simulink model "admire_linear_test"  (Simulink 3.00)
settings: Solver=ode4  StartTime=0.0  StopTime=30  FixedStep=0.008  RelTol=1e-3
undefined symbols (not defined in the file or in its folder): Abare, Afcs, Alt, Bbare, Bfcs, Cbare, Cfcs, dalt_err, Dbare, ddc_bw, ddc_rate, ddei_bw, ddei_rate, ddey_bw, ddey_rate, ddle_bw, ddle_rate, ddr_bw, ddr_rate, Dfcs, dMach_err, Mach, rlimit_c, rlimit_ie, rlimit_le, rlimit_oe, rlimit_r, y0bare
libraries: simulink_extras x16
settings Model: TimeSaveName=tout_lin  OutputSaveName=yout_lin  LastModifiedBy=hkg

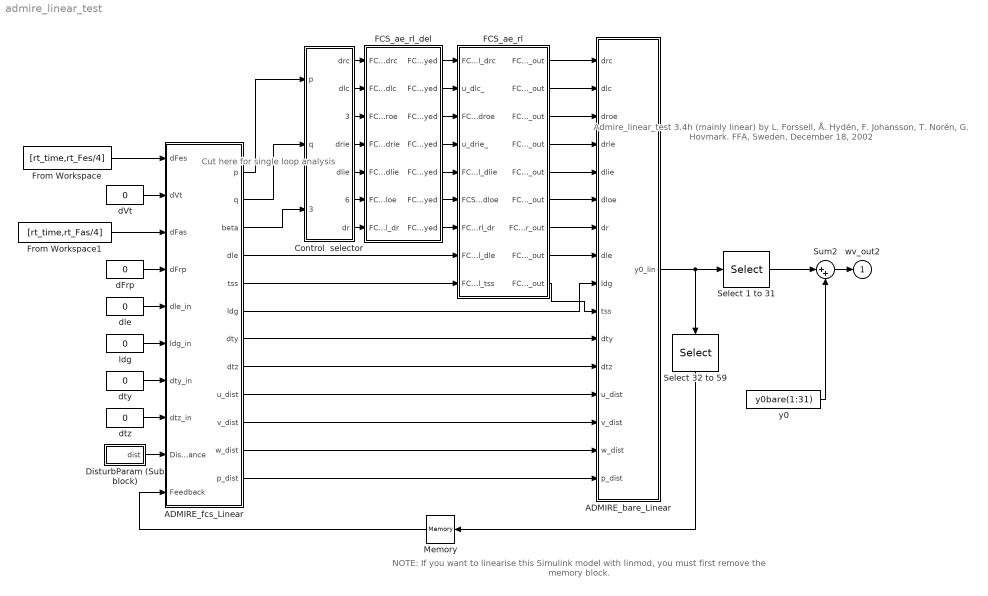
== system admire_linear_test ==
  note: Admire_linear_test 3.4h
      | (mainly linear)
      | by  L. Forssell,
      | Å. Hydén,
      | F. Johansson,
      | T. Norén,
      | G. Hovmark.
      | FFA, Sweden,
      | December 18, 2002
  note: Cut
      | here
      | for
      | single
      | loop
      | analysis
  note: NOTE: If you want to linearise this Simulink model
      | with linmod, you must first
      | remove the memory block.
  ADMIRE_bare_Linear : Subsystem
  ADMIRE_fcs_Linear : Subsystem
  Control  selector : Subsystem
  DisturbParam (Sub block) : Subsystem
  FCS_ae_rl : Subsystem
      mask Display: disp('Saturators,\nRatelimiters\nand\nActuators\n\nMach No and\nrate limiter\ndata are\ntaken from\nWorkspace\n\nAll inital\nstates empty')
  FCS_ae_rl_del : Subsystem
      mask Display: disp('Total\nComputer\nDelay\n\nAll inital\nstates empty')
  From Workspace : FromWorkspace  VariableName=[rt_time,rt_Fes/4]  SampleTime=0  HoldFinalValue=off
  From Workspace1 : FromWorkspace  VariableName=[rt_time,rt_Fas/4]  SampleTime=0  HoldFinalValue=off
  Memory : Memory  Orientation=left  X0=0  InheritSampleTime=off
  Select 1 to 31 : Selector  Elements=[1:31]  InputPortWidth=59
  Select 32 to 59 : Selector  Orientation=down  Elements=[32:59]  InputPortWidth=59
  Sum2 : Sum  Inputs=|++  SaturateOnIntegerOverflow=on
  dFrp : Constant  Value=0
  dVt : Constant  Value=0
  dle : Constant  Value=0
  dty : Constant  Value=0
  dtz : Constant  Value=0
  ldg : Constant  Value=0
  y0 : Constant  Value=y0bare(1:31)
  wv_out2 : Outport  Port=1  InitialOutput=0
  wires:
  dle/1 -> ADMIRE_fcs_Linear/5(dle_in)
  ldg/1 -> ADMIRE_fcs_Linear/6(ldg_in)
  dty/1 -> ADMIRE_fcs_Linear/7(dty_in)
  dtz/1 -> ADMIRE_fcs_Linear/8(dtz_in)
  DisturbParam (Sub block)/1(dist) -> ADMIRE_fcs_Linear/9(Disturbance)
  dFrp/1 -> ADMIRE_fcs_Linear/4(dFrp)
  dVt/1 -> ADMIRE_fcs_Linear/2(dVt)
  ADMIRE_fcs_Linear/12(p_dist) -> ADMIRE_bare_Linear/16(p_dist)
  ADMIRE_fcs_Linear/8(dtz) -> ADMIRE_bare_Linear/12(dtz)
  ADMIRE_fcs_Linear/7(dty) -> ADMIRE_bare_Linear/11(dty)
  FCS_ae_rl_del/1(FCS_ae_rl_del_drc_delayed) -> FCS_ae_rl/1(FCS_ae_rl_drc)
  FCS_ae_rl_del/2(FCS_ae_rl_del_dlc_delayed) -> FCS_ae_rl/2(u_dlc_)
  FCS_ae_rl_del/3(FCS_ae_rl_del_droe_delayed) -> FCS_ae_rl/3(FCS_ae_rl_droe)
  FCS_ae_rl_del/4(FCS_ae_rl_del_drie_delayed) -> FCS_ae_rl/4(u_drie_)
  FCS_ae_rl_del/5(FCS_ae_rl_del_dlie_delayed) -> FCS_ae_rl/5(FCS_ae_rl_dlie)
  FCS_ae_rl_del/6(FCS_ae_rl_del_dloe_delayed) -> FCS_ae_rl/6(FCS_ae_rl_dloe)
  FCS_ae_rl_del/7(FCS_ae_rl_del_dr_delayed) -> FCS_ae_rl/7(FCS_ae_rl_dr)
  ADMIRE_fcs_Linear/4(dle) -> FCS_ae_rl/8(FCS_ae_rl_dle)
  ADMIRE_fcs_Linear/5(tss) -> FCS_ae_rl/9(FCS_ae_rl_tss)
  ADMIRE_fcs_Linear/6(ldg) -> ADMIRE_bare_Linear/9(ldg)
  ADMIRE_fcs_Linear/9(u_dist) -> ADMIRE_bare_Linear/13(u_dist)
  ADMIRE_fcs_Linear/10(v_dist) -> ADMIRE_bare_Linear/14(v_dist)
  ADMIRE_fcs_Linear/11(w_dist) -> ADMIRE_bare_Linear/15(w_dist)
  FCS_ae_rl/1(FCS_ae_rl_drc_out) -> ADMIRE_bare_Linear/1(drc)
  FCS_ae_rl/2(FCS_ae_rl_dlc_out) -> ADMIRE_bare_Linear/2(dlc)
  FCS_ae_rl/3(FCS_ae_rl_droe_out) -> ADMIRE_bare_Linear/3(droe)
  FCS_ae_rl/4(FCS_ae_rl_drie_out) -> ADMIRE_bare_Linear/4(drie)
  FCS_ae_rl/5(FCS_ae_rl_dlie_out) -> ADMIRE_bare_Linear/5(dlie)
  FCS_ae_rl/6(FCS_ae_rl_dloe_out) -> ADMIRE_bare_Linear/6(dloe)
  FCS_ae_rl/7(FCS_ae_rl_dr_out) -> ADMIRE_bare_Linear/7(dr)
  FCS_ae_rl/8(FCS_ae_rl_dle_out) -> ADMIRE_bare_Linear/8(dle)
  FCS_ae_rl/9(FCS_ae_rl_tss_out) -> ADMIRE_bare_Linear/10(tss)
  ADMIRE_bare_Linear/1(y0_lin) -> Select 1 to 31/1, Select 32 to 59/1
  Select 32 to 59/1 -> Memory/1
  Sum2/1 -> wv_out2/1
  y0/1 -> Sum2/2
  Select 1 to 31/1 -> Sum2/1
  Memory/1 -> ADMIRE_fcs_Linear/10(Feedback)
  Control  selector/1(drc) -> FCS_ae_rl_del/1(FCS_ae_rl_del_drc)
  Control  selector/2(dlc) -> FCS_ae_rl_del/2(FCS_ae_rl_del_dlc)
  Control  selector/3(droe) -> FCS_ae_rl_del/3(FCS_ae_rl_del_droe)
  Control  selector/4(drie) -> FCS_ae_rl_del/4(FCS_ae_rl_del_drie)
  Control  selector/5(dlie) -> FCS_ae_rl_del/5(FCS_ae_rl_del_dlie)
  Control  selector/6(dloe) -> FCS_ae_rl_del/6(FCS_ae_rl_del_dloe)
  Control  selector/7(dr) -> FCS_ae_rl_del/7(FCS_ae_rl_del_dr)
  ADMIRE_fcs_Linear/1(p) -> Control  selector/1(p)
  ADMIRE_fcs_Linear/2(q) -> Control  selector/2(q)
  ADMIRE_fcs_Linear/3(beta) -> Control  selector/3(beta)
  From Workspace/1 -> ADMIRE_fcs_Linear/1(dFes)
  From Workspace1/1 -> ADMIRE_fcs_Linear/3(dFas)

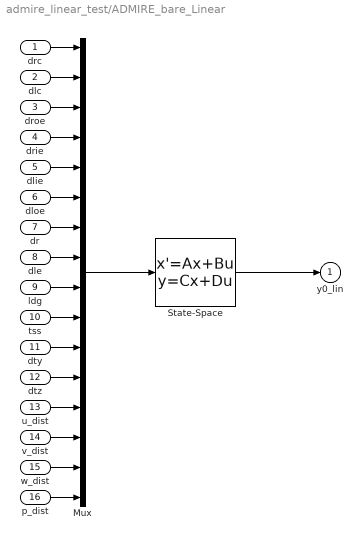
== system admire_linear_test/ADMIRE_bare_Linear ==
  drc : Inport  Port=1  PortWidth=-1  SampleTime=-1  DataType=auto
      settings: SignalType=auto
  dlc : Inport  Port=2  PortWidth=-1  SampleTime=-1  DataType=auto
      settings: SignalType=auto
  droe : Inport  Port=3  PortWidth=-1  SampleTime=-1  DataType=auto
      settings: SignalType=auto
  drie : Inport  Port=4  PortWidth=-1  SampleTime=-1  DataType=auto
      settings: SignalType=auto
  dlie : Inport  Port=5  PortWidth=-1  SampleTime=-1  DataType=auto
      settings: SignalType=auto
  dloe : Inport  Port=6  PortWidth=-1  SampleTime=-1  DataType=auto
      settings: SignalType=auto
  dr : Inport  Port=7  PortWidth=-1  SampleTime=-1  DataType=auto
      settings: SignalType=auto
  dle : Inport  Port=8  PortWidth=-1  SampleTime=-1  DataType=auto
      settings: SignalType=auto
  ldg : Inport  Port=9  PortWidth=-1  SampleTime=-1  DataType=auto
      settings: SignalType=auto
  tss : Inport  Port=10  PortWidth=-1  SampleTime=-1  DataType=auto
      settings: SignalType=auto
  dty : Inport  Port=11  PortWidth=-1  SampleTime=-1  DataType=auto
      settings: SignalType=auto
  dtz : Inport  Port=12  PortWidth=-1  SampleTime=-1  DataType=auto
      settings: SignalType=auto
  u_dist : Inport  Port=13  PortWidth=-1  SampleTime=-1  DataType=auto
      settings: SignalType=auto
  v_dist : Inport  Port=14  PortWidth=-1  SampleTime=-1  DataType=auto
      settings: SignalType=auto
  w_dist : Inport  Port=15  PortWidth=-1  SampleTime=-1  DataType=auto
      settings: SignalType=auto
  p_dist : Inport  Port=16  PortWidth=-1  SampleTime=-1  DataType=auto
      settings: SignalType=auto
  Mux : Mux  Inputs=16
      settings: DisplayOption=none
  State-Space : StateSpace  A=Abare  B=Bbare  C=Cbare  D=Dbare  X0=[]
  y0_lin : Outport  Port=1  InitialOutput=0
  wires:
  w_dist/1 -> Mux/15
  p_dist/1 -> Mux/16
  drc/1 -> Mux/1
  dlc/1 -> Mux/2
  droe/1 -> Mux/3
  drie/1 -> Mux/4
  dlie/1 -> Mux/5
  dloe/1 -> Mux/6
  dr/1 -> Mux/7
  dle/1 -> Mux/8
  ldg/1 -> Mux/9
  tss/1 -> Mux/10
  dty/1 -> Mux/11
  dtz/1 -> Mux/12
  u_dist/1 -> Mux/13
  v_dist/1 -> Mux/14
  Mux/1 -> State-Space/1
  State-Space/1 -> y0_lin/1

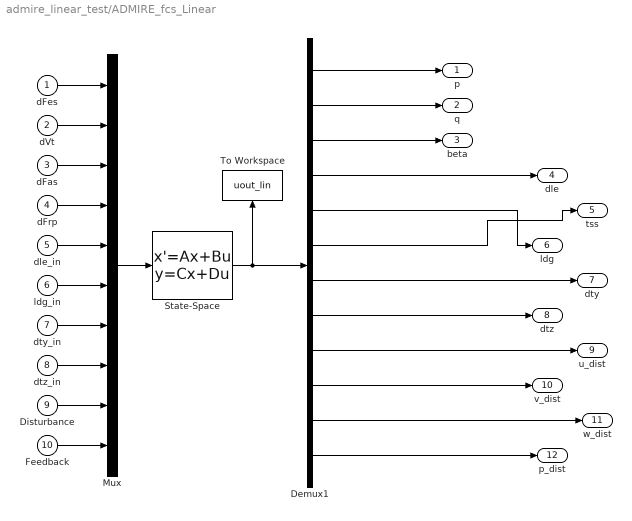
== system admire_linear_test/ADMIRE_fcs_Linear ==
  dFes : Inport  Port=1  PortWidth=-1  SampleTime=-1  DataType=auto
      settings: SignalType=auto
  dVt : Inport  Port=2  PortWidth=-1  SampleTime=-1  DataType=auto
      settings: SignalType=auto
  dFas : Inport  Port=3  PortWidth=-1  SampleTime=-1  DataType=auto
      settings: SignalType=auto
  dFrp : Inport  Port=4  PortWidth=-1  SampleTime=-1  DataType=auto
      settings: SignalType=auto
  dle_in : Inport  Port=5  PortWidth=-1  SampleTime=-1  DataType=auto
      settings: SignalType=auto
  ldg_in : Inport  Port=6  PortWidth=-1  SampleTime=-1  DataType=auto
      settings: SignalType=auto
  dty_in : Inport  Port=7  PortWidth=-1  SampleTime=-1  DataType=auto
      settings: SignalType=auto
  dtz_in : Inport  Port=8  PortWidth=-1  SampleTime=-1  DataType=auto
      settings: SignalType=auto
  Disturbance : Inport  Port=9  PortWidth=-1  SampleTime=-1  DataType=auto
      settings: SignalType=auto
  Feedback : Inport  Port=10  PortWidth=-1  SampleTime=-1  DataType=auto
      settings: SignalType=auto
  Demux1 : Demux  Outputs=12
  Mux : Mux  Inputs=10
  State-Space : StateSpace  A=Afcs  B=Bfcs  C=Cfcs  D=Dfcs  X0=[]
  To Workspace : ToWorkspace  VariableName=uout_lin  SampleTime=-1  SaveFormat=Matrix
      settings: Orientation=up
  p : Outport  Port=1
  q : Outport  Port=2
  beta : Outport  Port=3
  dle : Outport  Port=4
  tss : Outport  Port=5
  ldg : Outport  Port=6
  dty : Outport  Port=7
  dtz : Outport  Port=8
  u_dist : Outport  Port=9
  v_dist : Outport  Port=10
  w_dist : Outport  Port=11
  p_dist : Outport  Port=12
  wires:
  State-Space/1 -> Demux1/1, To Workspace/1
  Mux/1 -> State-Space/1
  dFes/1 -> Mux/1
  dVt/1 -> Mux/2
  dFas/1 -> Mux/3
  dFrp/1 -> Mux/4
  dle_in/1 -> Mux/5
  ldg_in/1 -> Mux/6
  dty_in/1 -> Mux/7
  dtz_in/1 -> Mux/8
  Disturbance/1 -> Mux/9
  Feedback/1 -> Mux/10
  Demux1/3 -> beta/1
  Demux1/2 -> q/1
  Demux1/1 -> p/1
  Demux1/4 -> dle/1
  Demux1/7 -> dty/1
  Demux1/12 -> p_dist/1
  Demux1/11 -> w_dist/1
  Demux1/10 -> v_dist/1
  Demux1/9 -> u_dist/1
  Demux1/8 -> dtz/1
  Demux1/5 -> ldg/1
  Demux1/6 -> tss/1

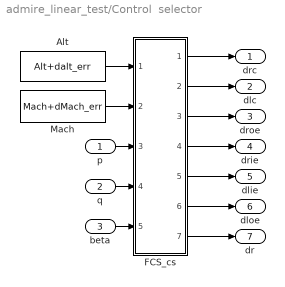
== system admire_linear_test/Control  selector ==
  p : Inport  Port=1  PortWidth=-1  SampleTime=-1  DataType=auto
      settings: SignalType=auto
  q : Inport  Port=2  PortWidth=-1  SampleTime=-1  DataType=auto
      settings: SignalType=auto
  beta : Inport  Port=3  PortWidth=-1  SampleTime=-1  DataType=auto
      settings: SignalType=auto
  Alt : Constant  Value=Alt+dalt_err
  "FCS_cs " : Subsystem
      mask Display: disp('FCS_cs')
  Mach : Constant  Value=Mach+dMach_err
  drc : Outport  Port=1
  dlc : Outport  Port=2
  droe : Outport  Port=3
  drie : Outport  Port=4
  dlie : Outport  Port=5
  dloe : Outport  Port=6
  dr : Outport  Port=7
  wires:
  Alt/1 -> "FCS_cs "/1(FCS_cs_Altitude)
  Mach/1 -> "FCS_cs "/2(FCS_cs_Mach)
  "FCS_cs "/1(FCS_cs_drc) -> drc/1
  "FCS_cs "/2(FCS_cs_dlc) -> dlc/1
  "FCS_cs "/3(FCS_cs_droe) -> droe/1
  "FCS_cs "/4(FCS_cs_drie) -> drie/1
  p/1 -> "FCS_cs "/3(FCS_cs_p)
  "FCS_cs "/5(FCS_cs_dlie) -> dlie/1
  q/1 -> "FCS_cs "/4(FCS_cs_q)
  "FCS_cs "/6(FCS_cs_dloe) -> dloe/1
  beta/1 -> "FCS_cs "/5(FCS_cs_beta)
  "FCS_cs "/7(FCS_cs_dr) -> dr/1

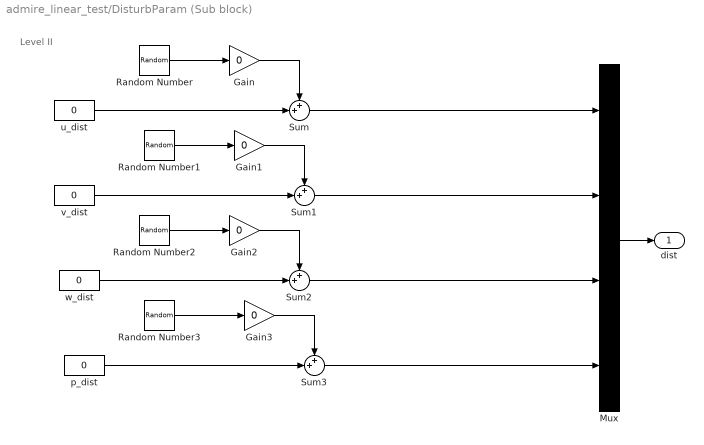
== system admire_linear_test/DisturbParam (Sub block) ==
  note: Level II
  Gain{,1..3} (4 alike) : Gain  Gain=0  SaturateOnIntegerOverflow=on
  Mux : Mux  Inputs=4
      settings: DisplayOption=none
  Random Number : RandomNumber  Mean=0  Variance=1  Seed=1  SampleTime=0
  Random Number1 : RandomNumber  Mean=0  Variance=1  Seed=2  SampleTime=0
  Random Number2 : RandomNumber  Mean=0  Variance=1  Seed=3  SampleTime=0
  Random Number3 : RandomNumber  Mean=0  Variance=1  Seed=4  SampleTime=0
  Sum{,1..3} (4 alike) : Sum  Inputs=++|  SaturateOnIntegerOverflow=on
  "p_dist " : Constant  Value=0
  "u_dist " : Constant  Value=0
  "v_dist " : Constant  Value=0
  "w_dist " : Constant  Value=0
  dist : Outport  Port=1
  wires:
  Mux/1 -> dist/1
  "u_dist "/1 -> Sum/2
  Gain/1 -> Sum/1
  Random Number/1 -> Gain/1
  Sum/1 -> Mux/1
  "v_dist "/1 -> Sum1/2
  Gain1/1 -> Sum1/1
  Random Number1/1 -> Gain1/1
  Sum1/1 -> Mux/2
  "w_dist "/1 -> Sum2/2
  Gain2/1 -> Sum2/1
  Random Number2/1 -> Gain2/1
  Sum2/1 -> Mux/3
  "p_dist "/1 -> Sum3/2
  Gain3/1 -> Sum3/1
  Random Number3/1 -> Gain3/1
  Sum3/1 -> Mux/4

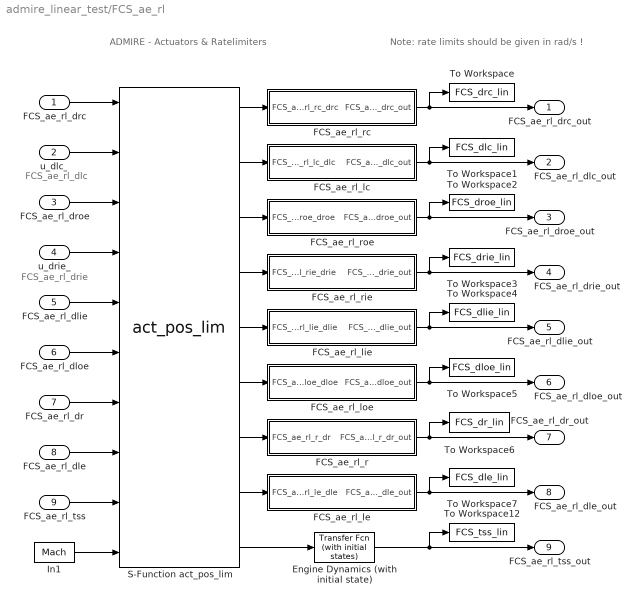
== system admire_linear_test/FCS_ae_rl ==
  note: Note: rate limits should be given
      | in rad/s !
  note: FCS_ae_rl_dlc
  note: FCS_ae_rl_drie
  note: ADMIRE - Actuators & Ratelimiters
  FCS_ae_rl_drc : Inport  Port=1  PortWidth=-1  SampleTime=-1  DataType=auto
      settings: SignalType=auto
  u_dlc_ : Inport  Port=2  PortWidth=-1  SampleTime=-1  DataType=auto
      settings: SignalType=auto
  FCS_ae_rl_droe : Inport  Port=3  PortWidth=-1  SampleTime=-1  DataType=auto
      settings: SignalType=auto
  u_drie_ : Inport  Port=4  PortWidth=-1  SampleTime=-1  DataType=auto
      settings: SignalType=auto
  FCS_ae_rl_dlie : Inport  Port=5  PortWidth=-1  SampleTime=-1  DataType=auto
      settings: SignalType=auto
  FCS_ae_rl_dloe : Inport  Port=6  PortWidth=-1  SampleTime=-1  DataType=auto
      settings: SignalType=auto
  FCS_ae_rl_dr : Inport  Port=7  PortWidth=-1  SampleTime=-1  DataType=auto
      settings: SignalType=auto
  FCS_ae_rl_dle : Inport  Port=8  PortWidth=-1  SampleTime=-1  DataType=auto
      settings: SignalType=auto
  FCS_ae_rl_tss : Inport  Port=9  PortWidth=-1  SampleTime=-1  DataType=auto
      settings: SignalType=auto
  Engine Dynamics (with initial state) : simulink_extras/Additional Linear/Transfer Fcn (with initial states)  N=[1]  D="[2  1]"  X0=[0]
  FCS_ae_rl_lc : Subsystem
      mask Display: disp(' Ratelimiter and Dynamics\nServo: lc')
  FCS_ae_rl_le : Subsystem
      mask Display: disp(' Ratelimiter and Dynamics\nServo: le')
  FCS_ae_rl_lie : Subsystem
      mask Display: disp(' Ratelimiter and Dynamics\nServo: lie')
  FCS_ae_rl_loe : Subsystem
      mask Display: disp(' Ratelimiter and Dynamics\nServo: loe')
  FCS_ae_rl_r : Subsystem
      mask Display: disp(' Ratelimiter and Dynamics\nServo: r')
  FCS_ae_rl_rc : Subsystem
      mask Display: disp(' Ratelimiter and Dynamics\nServo: rc')
  FCS_ae_rl_rie : Subsystem
      mask Display: disp(' Ratelimiter and Dynamics\nServo: rie')
  FCS_ae_rl_roe : Subsystem
      mask Display: disp(' Ratelimiter and Dynamics\nServo: roe')
  In1 : Constant  Value=Mach
  S-Function act_pos_lim : S-Function  FunctionName=act_pos_lim  PortCounts=[]  SFunctionModules=''
      mask Display:
      | plot([-30 30],[-30 30])
      | plot([0 0],[-30 30])
      | plot([-50 50],[0 0])
      | plot([30 50],[30 30])
      | plot([-50 -30],[-30 -30])
      | plot([-5 0],[25 30])
      | plot([5 0],[25 30])
      | plot([45 50],[3 0])
      | plot([45 50],[-3 0])
      | text(-21,26,'out')
      | text(30,-2,'in')
  To Workspace : ToWorkspace  VariableName=FCS_drc_lin  SampleTime=-1  SaveFormat=Matrix
  To Workspace1 : ToWorkspace  VariableName=FCS_dlc_lin  SampleTime=-1  SaveFormat=Matrix
  To Workspace12 : ToWorkspace  VariableName=FCS_tss_lin  SampleTime=-1  SaveFormat=Matrix
  To Workspace2 : ToWorkspace  VariableName=FCS_droe_lin  SampleTime=-1  SaveFormat=Matrix
  To Workspace3 : ToWorkspace  VariableName=FCS_drie_lin  SampleTime=-1  SaveFormat=Matrix
  To Workspace4 : ToWorkspace  VariableName=FCS_dlie_lin  SampleTime=-1  SaveFormat=Matrix
  To Workspace5 : ToWorkspace  VariableName=FCS_dloe_lin  SampleTime=-1  SaveFormat=Matrix
  To Workspace6 : ToWorkspace  VariableName=FCS_dr_lin  SampleTime=-1  SaveFormat=Matrix
  To Workspace7 : ToWorkspace  VariableName=FCS_dle_lin  SampleTime=-1  SaveFormat=Matrix
  FCS_ae_rl_drc_out : Outport  Port=1
  FCS_ae_rl_dlc_out : Outport  Port=2
  FCS_ae_rl_droe_out : Outport  Port=3
  FCS_ae_rl_drie_out : Outport  Port=4
  FCS_ae_rl_dlie_out : Outport  Port=5
  FCS_ae_rl_dloe_out : Outport  Port=6
  FCS_ae_rl_dr_out : Outport  Port=7
  FCS_ae_rl_dle_out : Outport  Port=8
  FCS_ae_rl_tss_out : Outport  Port=9
  wires:
  S-Function act_pos_lim/2 -> FCS_ae_rl_lc/1(FCS_ae_rl_lc_dlc)
  S-Function act_pos_lim/3 -> FCS_ae_rl_roe/1(FCS_ae_rl_roe_droe)
  S-Function act_pos_lim/5 -> FCS_ae_rl_lie/1(FCS_ae_rl_lie_dlie)
  S-Function act_pos_lim/6 -> FCS_ae_rl_loe/1(FCS_ae_rl_loe_dloe)
  S-Function act_pos_lim/7 -> FCS_ae_rl_r/1(FCS_ae_rl_r_dr)
  S-Function act_pos_lim/8 -> FCS_ae_rl_le/1(FCS_ae_rl_le_dle)
  S-Function act_pos_lim/9 -> Engine Dynamics (with initial state)/1
  S-Function act_pos_lim/1 -> FCS_ae_rl_rc/1(FCS_ae_rl_rc_drc)
  S-Function act_pos_lim/4 -> FCS_ae_rl_rie/1(FCS_ae_rl_rie_drie)
  In1/1 -> S-Function act_pos_lim/10
  u_dlc_/1 -> S-Function act_pos_lim/2
  FCS_ae_rl_drc/1 -> S-Function act_pos_lim/1
  FCS_ae_rl_droe/1 -> S-Function act_pos_lim/3
  FCS_ae_rl_dlie/1 -> S-Function act_pos_lim/5
  FCS_ae_rl_dloe/1 -> S-Function act_pos_lim/6
  FCS_ae_rl_dr/1 -> S-Function act_pos_lim/7
  u_drie_/1 -> S-Function act_pos_lim/4
  FCS_ae_rl_dle/1 -> S-Function act_pos_lim/8
  FCS_ae_rl_tss/1 -> S-Function act_pos_lim/9
  FCS_ae_rl_rc/1(FCS_ae_rl_rc_drc_out) -> To Workspace/1, FCS_ae_rl_drc_out/1
  FCS_ae_rl_lc/1(FCS_ae_rl_lc_dlc_out) -> To Workspace1/1, FCS_ae_rl_dlc_out/1
  Engine Dynamics (with initial state)/1 -> To Workspace12/1, FCS_ae_rl_tss_out/1
  FCS_ae_rl_le/1(FCS_ae_rl_le_dle_out) -> To Workspace7/1, FCS_ae_rl_dle_out/1
  FCS_ae_rl_r/1(FCS_ae_rl_r_dr_out) -> To Workspace6/1, FCS_ae_rl_dr_out/1
  FCS_ae_rl_loe/1(FCS_ae_rl_loe_dloe_out) -> To Workspace5/1, FCS_ae_rl_dloe_out/1
  FCS_ae_rl_lie/1(FCS_ae_rl_lie_dlie_out) -> To Workspace4/1, FCS_ae_rl_dlie_out/1
  FCS_ae_rl_roe/1(FCS_ae_rl_roe_droe_out) -> To Workspace2/1, FCS_ae_rl_droe_out/1
  FCS_ae_rl_rie/1(FCS_ae_rl_rie_drie_out) -> To Workspace3/1, FCS_ae_rl_drie_out/1

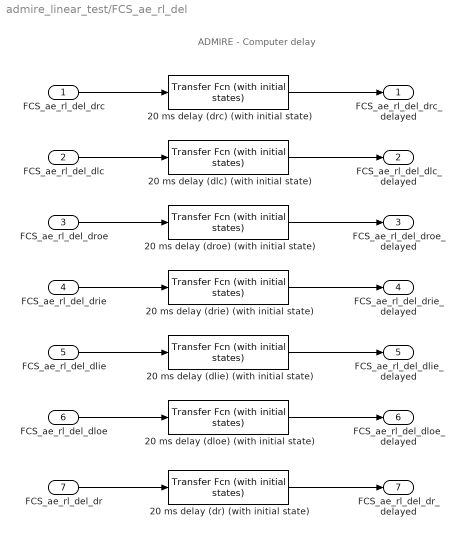
== system admire_linear_test/FCS_ae_rl_del ==
  note: ADMIRE - Computer delay
  FCS_ae_rl_del_drc : Inport  Port=1  PortWidth=-1  SampleTime=-1  DataType=auto
      settings: SignalType=auto
  FCS_ae_rl_del_dlc : Inport  Port=2  PortWidth=-1  SampleTime=-1  DataType=auto
      settings: SignalType=auto
  FCS_ae_rl_del_droe : Inport  Port=3  PortWidth=-1  SampleTime=-1  DataType=auto
      settings: SignalType=auto
  FCS_ae_rl_del_drie : Inport  Port=4  PortWidth=-1  SampleTime=-1  DataType=auto
      settings: SignalType=auto
  FCS_ae_rl_del_dlie : Inport  Port=5  PortWidth=-1  SampleTime=-1  DataType=auto
      settings: SignalType=auto
  FCS_ae_rl_del_dloe : Inport  Port=6  PortWidth=-1  SampleTime=-1  DataType=auto
      settings: SignalType=auto
  FCS_ae_rl_del_dr : Inport  Port=7  PortWidth=-1  SampleTime=-1  DataType=auto
      settings: SignalType=auto
  20 ms delay (dlc) (with initial state) : simulink_extras/Additional Linear/Transfer Fcn (with initial states)  N=[0.000033 -0.01 1]  D=[0.000033 0.01 1]  X0=[]
  20 ms delay (dlie) (with initial state) : simulink_extras/Additional Linear/Transfer Fcn (with initial states)  N=[0.000033 -0.01 1]  D=[0.000033 0.01 1]  X0=[]
  20 ms delay (dloe) (with initial state) : simulink_extras/Additional Linear/Transfer Fcn (with initial states)  N=[0.000033 -0.01 1]  D=[0.000033 0.01 1]  X0=[]
  20 ms delay (dr) (with initial state) : simulink_extras/Additional Linear/Transfer Fcn (with initial states)  N=[0.000033 -0.01 1]  D=[0.000033 0.01 1]  X0=[]
  20 ms delay (drc) (with initial state) : simulink_extras/Additional Linear/Transfer Fcn (with initial states)  N=[0.000033 -0.01 1]  D=[0.000033 0.01 1]  X0=[]
  20 ms delay (drie) (with initial state) : simulink_extras/Additional Linear/Transfer Fcn (with initial states)  N=[0.000033 -0.01 1]  D=[0.000033 0.01 1]  X0=[]
  20 ms delay (droe) (with initial state) : simulink_extras/Additional Linear/Transfer Fcn (with initial states)  N=[0.000033 -0.01 1]  D=[0.000033 0.01 1]  X0=[]
  FCS_ae_rl_del_drc_delayed : Outport  Port=1
  FCS_ae_rl_del_dlc_delayed : Outport  Port=2
  FCS_ae_rl_del_droe_delayed : Outport  Port=3
  FCS_ae_rl_del_drie_delayed : Outport  Port=4
  FCS_ae_rl_del_dlie_delayed : Outport  Port=5
  FCS_ae_rl_del_dloe_delayed : Outport  Port=6
  FCS_ae_rl_del_dr_delayed : Outport  Port=7
  wires:
  FCS_ae_rl_del_drc/1 -> 20 ms delay (drc) (with initial state)/1
  FCS_ae_rl_del_dlc/1 -> 20 ms delay (dlc) (with initial state)/1
  FCS_ae_rl_del_droe/1 -> 20 ms delay (droe) (with initial state)/1
  FCS_ae_rl_del_drie/1 -> 20 ms delay (drie) (with initial state)/1
  FCS_ae_rl_del_dlie/1 -> 20 ms delay (dlie) (with initial state)/1
  FCS_ae_rl_del_dloe/1 -> 20 ms delay (dloe) (with initial state)/1
  FCS_ae_rl_del_dr/1 -> 20 ms delay (dr) (with initial state)/1
  20 ms delay (drc) (with initial state)/1 -> FCS_ae_rl_del_drc_delayed/1
  20 ms delay (dlc) (with initial state)/1 -> FCS_ae_rl_del_dlc_delayed/1
  20 ms delay (droe) (with initial state)/1 -> FCS_ae_rl_del_droe_delayed/1
  20 ms delay (drie) (with initial state)/1 -> FCS_ae_rl_del_drie_delayed/1
  20 ms delay (dlie) (with initial state)/1 -> FCS_ae_rl_del_dlie_delayed/1
  20 ms delay (dloe) (with initial state)/1 -> FCS_ae_rl_del_dloe_delayed/1
  20 ms delay (dr) (with initial state)/1 -> FCS_ae_rl_del_dr_delayed/1

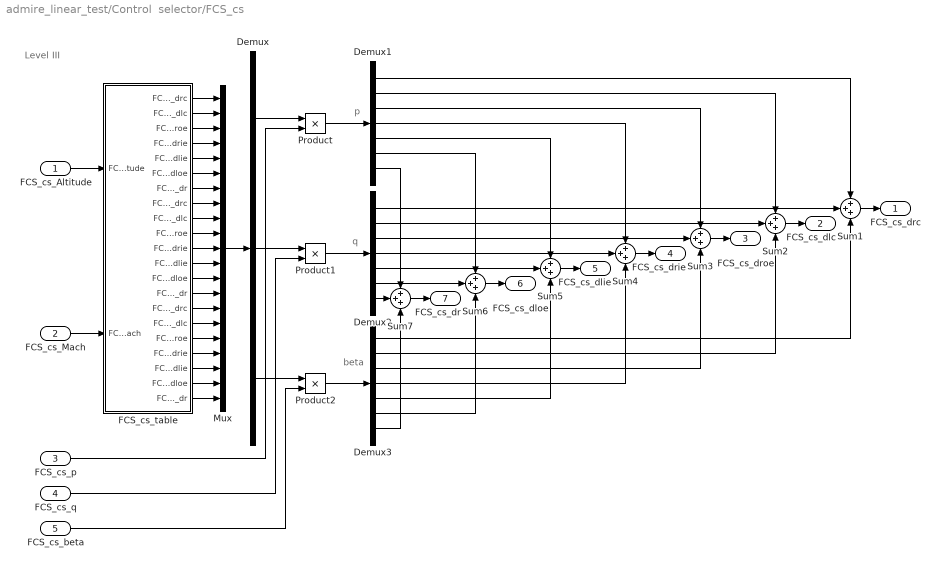
== system admire_linear_test/Control  selector/FCS_cs  ==
  note: p
  note: q
  note: beta
  note: Level III
  FCS_cs_Altitude : Inport  Port=1  PortWidth=-1  SampleTime=-1  DataType=auto
      settings: SignalType=auto
  FCS_cs_Mach : Inport  Port=2  PortWidth=-1  SampleTime=-1  DataType=auto
      settings: SignalType=auto
  FCS_cs_p : Inport  Port=3  PortWidth=-1  SampleTime=-1  DataType=auto
      settings: SignalType=auto
  FCS_cs_q : Inport  Port=4  PortWidth=-1  SampleTime=-1  DataType=auto
      settings: SignalType=auto
  FCS_cs_beta : Inport  Port=5  PortWidth=-1  SampleTime=-1  DataType=auto
      settings: SignalType=auto
  Demux : Demux  Outputs=[7 7 7]
  Demux1 : Demux  Outputs=7
  Demux2 : Demux  Outputs=7
  Demux3 : Demux  Outputs=7
  FCS_cs_table : Subsystem
      mask Display: disp('FCS_cs_table')
  Mux : Mux  Inputs=21
  Product : Product  Inputs=2  SaturateOnIntegerOverflow=on
  Product1 : Product  Inputs=2  SaturateOnIntegerOverflow=on
  Product2 : Product  Inputs=2  SaturateOnIntegerOverflow=on
  Sum{1..7} (7 alike) : Sum  Inputs=3  SaturateOnIntegerOverflow=on
  FCS_cs_drc : Outport  Port=1
  FCS_cs_dlc : Outport  Port=2
  FCS_cs_droe : Outport  Port=3
  FCS_cs_drie : Outport  Port=4
  FCS_cs_dlie : Outport  Port=5
  FCS_cs_dloe : Outport  Port=6
  FCS_cs_dr : Outport  Port=7
  wires:
  Mux/1 -> Demux/1
  Demux/1 -> Product/1
  Demux/2 -> Product1/1
  Demux/3 -> Product2/1
  FCS_cs_p/1 -> Product/2
  FCS_cs_q/1 -> Product1/2
  FCS_cs_beta/1 -> Product2/2
  FCS_cs_Altitude/1 -> FCS_cs_table/1(FCS_cs_table_Altitude)
  FCS_cs_Mach/1 -> FCS_cs_table/2(FCS_cs_table_Mach)
  FCS_cs_table/1(FCS_cs_table_p_drc) -> Mux/1
  FCS_cs_table/2(FCS_cs_table_p_dlc) -> Mux/2
  FCS_cs_table/3(FCS_cs_table_p_droe) -> Mux/3
  FCS_cs_table/4(FCS_cs_table_p_drie) -> Mux/4
  FCS_cs_table/5(FCS_cs_table_p_dlie) -> Mux/5
  FCS_cs_table/6(FCS_cs_table_p_dloe) -> Mux/6
  FCS_cs_table/7(FCS_cs_table_p_dr) -> Mux/7
  FCS_cs_table/8(FCS_cs_table_q_drc) -> Mux/8
  FCS_cs_table/9(FCS_cs_table_q_dlc) -> Mux/9
  FCS_cs_table/10(FCS_cs_table_q_droe) -> Mux/10
  FCS_cs_table/11(FCS_cs_table_q_drie) -> Mux/11
  FCS_cs_table/12(FCS_cs_table_q_dlie) -> Mux/12
  FCS_cs_table/14(FCS_cs_table_q_dr) -> Mux/14
  FCS_cs_table/13(FCS_cs_table_q_dloe) -> Mux/13
  FCS_cs_table/15(FCS_cs_table_beta_drc) -> Mux/15
  FCS_cs_table/16(FCS_cs_table_beta_dlc) -> Mux/16
  FCS_cs_table/17(FCS_cs_table_beta_droe) -> Mux/17
  FCS_cs_table/18(FCS_cs_table_beta_drie) -> Mux/18
  FCS_cs_table/19(FCS_cs_table_beta_dlie) -> Mux/19
  FCS_cs_table/20(FCS_cs_table_beta_dloe) -> Mux/20
  FCS_cs_table/21(FCS_cs_table_beta_dr) -> Mux/21
  Product/1 -> Demux1/1
  Product1/1 -> Demux2/1
  Product2/1 -> Demux3/1
  Demux2/6 -> Sum6/2
  Demux2/7 -> Sum7/2
  Demux1/7 -> Sum7/1
  Demux3/7 -> Sum7/3
  Sum7/1 -> FCS_cs_dr/1
  Demux2/5 -> Sum5/2
  Demux1/6 -> Sum6/1
  Demux3/6 -> Sum6/3
  Sum6/1 -> FCS_cs_dloe/1
  Demux2/4 -> Sum4/2
  Demux1/5 -> Sum5/1
  Demux3/5 -> Sum5/3
  Sum5/1 -> FCS_cs_dlie/1
  Demux2/3 -> Sum3/2
  Demux1/4 -> Sum4/1
  Demux3/4 -> Sum4/3
  Sum4/1 -> FCS_cs_drie/1
  Demux2/2 -> Sum2/2
  Demux1/3 -> Sum3/1
  Demux3/3 -> Sum3/3
  Sum3/1 -> FCS_cs_droe/1
  Demux2/1 -> Sum1/2
  Demux1/2 -> Sum2/1
  Demux3/2 -> Sum2/3
  Sum2/1 -> FCS_cs_dlc/1
  Demux1/1 -> Sum1/1
  Demux3/1 -> Sum1/3
  Sum1/1 -> FCS_cs_drc/1

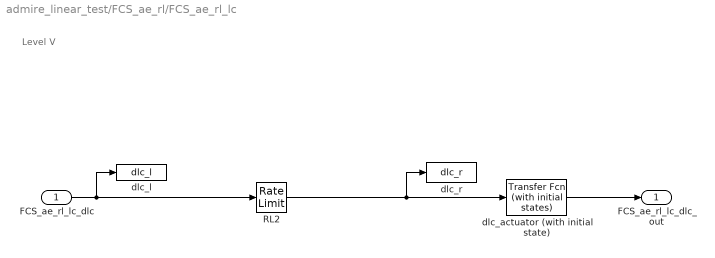
== system admire_linear_test/FCS_ae_rl/FCS_ae_rl_lc ==
  note: Level V
  FCS_ae_rl_lc_dlc : Inport  Port=1  PortWidth=-1  SampleTime=-1  DataType=auto
      settings: SignalType=auto
  RL2 : RateLimiter  RisingSlewLimit=rlimit_c+ddc_rate  FallingSlewLimit=-rlimit_c-ddc_rate
  dlc_actuator (with initial state) : simulink_extras/Additional Linear/Transfer Fcn (with initial states)  N=[1]  D="[0.05+ddc_bw  1]"  X0=[]
  dlc_l : ToWorkspace  VariableName=dlc_l  SampleTime=0  SaveFormat=Matrix
      settings: Buffer=10000
  dlc_r : ToWorkspace  VariableName=dlc_r  SampleTime=0  SaveFormat=Matrix
      settings: Buffer=10000
  FCS_ae_rl_lc_dlc_out : Outport  Port=1  InitialOutput=0
  wires:
  FCS_ae_rl_lc_dlc/1 -> dlc_l/1, RL2/1
  dlc_actuator (with initial state)/1 -> FCS_ae_rl_lc_dlc_out/1
  RL2/1 -> dlc_r/1, dlc_actuator (with initial state)/1

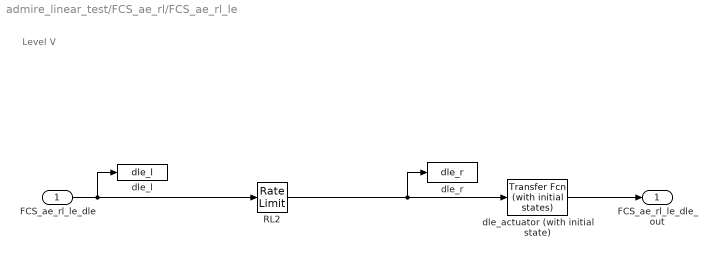
== system admire_linear_test/FCS_ae_rl/FCS_ae_rl_le ==
  note: Level V
  FCS_ae_rl_le_dle : Inport  Port=1  PortWidth=-1  SampleTime=-1  DataType=auto
      settings: SignalType=auto
  RL2 : RateLimiter  RisingSlewLimit=rlimit_le+ddle_rate  FallingSlewLimit=-rlimit_le-ddle_rate
  dle_actuator (with initial state) : simulink_extras/Additional Linear/Transfer Fcn (with initial states)  N=[1]  D="[0.05+ddle_bw  1]"  X0=[0]
  dle_l : ToWorkspace  VariableName=dle_l  SampleTime=0  SaveFormat=Matrix
      settings: Buffer=10000
  dle_r : ToWorkspace  VariableName=dle_r  SampleTime=0  SaveFormat=Matrix
      settings: Buffer=10000
  FCS_ae_rl_le_dle_out : Outport  Port=1  InitialOutput=0
  wires:
  FCS_ae_rl_le_dle/1 -> dle_l/1, RL2/1
  dle_actuator (with initial state)/1 -> FCS_ae_rl_le_dle_out/1
  RL2/1 -> dle_r/1, dle_actuator (with initial state)/1

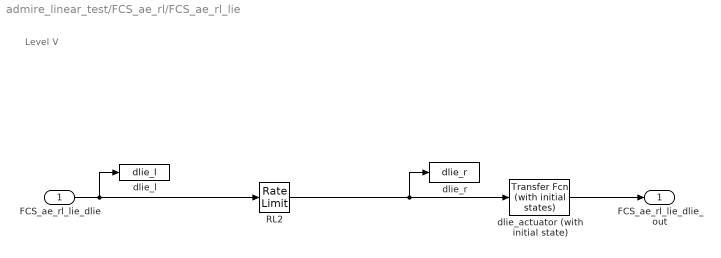
== system admire_linear_test/FCS_ae_rl/FCS_ae_rl_lie ==
  note: Level V
  FCS_ae_rl_lie_dlie : Inport  Port=1  PortWidth=-1  SampleTime=-1  DataType=auto
      settings: SignalType=auto
  RL2 : RateLimiter  RisingSlewLimit=rlimit_ie+ddei_rate  FallingSlewLimit=-rlimit_ie-ddei_rate
  dlie_actuator (with initial state) : simulink_extras/Additional Linear/Transfer Fcn (with initial states)  N=[1]  D="[0.05+ddei_bw  1]"  X0=[0]
  dlie_l : ToWorkspace  VariableName=dlie_l  SampleTime=0  SaveFormat=Matrix
      settings: Buffer=10000
  dlie_r : ToWorkspace  VariableName=dlie_r  SampleTime=0  SaveFormat=Matrix
      settings: Buffer=10000
  FCS_ae_rl_lie_dlie_out : Outport  Port=1  InitialOutput=0
  wires:
  dlie_actuator (with initial state)/1 -> FCS_ae_rl_lie_dlie_out/1
  FCS_ae_rl_lie_dlie/1 -> dlie_l/1, RL2/1
  RL2/1 -> dlie_actuator (with initial state)/1, dlie_r/1

== system admire_linear_test/FCS_ae_rl/FCS_ae_rl_loe ==
  note: Level V
  FCS_ae_rl_loe_dloe : Inport  Port=1  PortWidth=-1  SampleTime=-1  DataType=auto
      settings: SignalType=auto
  RL2 : RateLimiter  RisingSlewLimit=rlimit_oe+ddey_rate  FallingSlewLimit=-rlimit_oe-ddey_rate
  dloe_actuator (with initial state) : simulink_extras/Additional Linear/Transfer Fcn (with initial states)  N=[1]  D="[0.05+ddey_bw  1]"  X0=[0]
  dloe_l : ToWorkspace  VariableName=dloe_l  SampleTime=0  SaveFormat=Matrix
      settings: Buffer=10000
  dloe_r : ToWorkspace  VariableName=dloe_r  SampleTime=0  SaveFormat=Matrix
      settings: Buffer=10000
  FCS_ae_rl_loe_dloe_out : Outport  Port=1  InitialOutput=0
  wires:
  FCS_ae_rl_loe_dloe/1 -> dloe_l/1, RL2/1
  dloe_actuator (with initial state)/1 -> FCS_ae_rl_loe_dloe_out/1
  RL2/1 -> dloe_r/1, dloe_actuator (with initial state)/1

== system admire_linear_test/FCS_ae_rl/FCS_ae_rl_r ==
  note: Level V
  FCS_ae_rl_r_dr : Inport  Port=1  PortWidth=-1  SampleTime=-1  DataType=auto
      settings: SignalType=auto
  RL2 : RateLimiter  RisingSlewLimit=rlimit_r+ddr_rate  FallingSlewLimit=-rlimit_r-ddr_rate
  dr_actuator (with initial state) : simulink_extras/Additional Linear/Transfer Fcn (with initial states)  N=[1]  D="[0.05+ddr_bw  1]"  X0=[0]
  dr_l : ToWorkspace  VariableName=dr_l  SampleTime=0  SaveFormat=Matrix
      settings: Buffer=10000
  dr_r : ToWorkspace  VariableName=dr_r  SampleTime=0  SaveFormat=Matrix
      settings: Buffer=10000
  FCS_ae_rl_r_dr_out : Outport  Port=1  InitialOutput=0
  wires:
  dr_actuator (with initial state)/1 -> FCS_ae_rl_r_dr_out/1
  FCS_ae_rl_r_dr/1 -> dr_l/1, RL2/1
  RL2/1 -> dr_actuator (with initial state)/1, dr_r/1

== system admire_linear_test/FCS_ae_rl/FCS_ae_rl_rc ==
  note: Level V
  FCS_ae_rl_rc_drc : Inport  Port=1  PortWidth=-1  SampleTime=-1  DataType=auto
      settings: SignalType=auto
  RL2 : RateLimiter  RisingSlewLimit=rlimit_c+ddc_rate  FallingSlewLimit=-rlimit_c-ddc_rate
  drc_actuator (with initial state) : simulink_extras/Additional Linear/Transfer Fcn (with initial states)  N=[1]  D="[0.05+ddc_bw  1]"  X0=[]
  drc_l : ToWorkspace  VariableName=drc_l  SampleTime=0  SaveFormat=Matrix
      settings: Buffer=10000
  drc_r : ToWorkspace  VariableName=drc_r  SampleTime=0  SaveFormat=Matrix
      settings: Buffer=10000
  FCS_ae_rl_rc_drc_out : Outport  Port=1  InitialOutput=0
  wires:
  drc_actuator (with initial state)/1 -> FCS_ae_rl_rc_drc_out/1
  FCS_ae_rl_rc_drc/1 -> drc_l/1, RL2/1
  RL2/1 -> drc_actuator (with initial state)/1, drc_r/1

== system admire_linear_test/FCS_ae_rl/FCS_ae_rl_rie ==
  note: Level V
  FCS_ae_rl_rie_drie : Inport  Port=1  PortWidth=-1  SampleTime=-1  DataType=auto
      settings: SignalType=auto
  RL2 : RateLimiter  RisingSlewLimit=rlimit_ie+ddei_rate  FallingSlewLimit=-rlimit_ie-ddei_rate
  drie_actuator (with initial state) : simulink_extras/Additional Linear/Transfer Fcn (with initial states)  N=[1]  D="[0.05+ddei_bw  1]"  X0=[]
  drie_l : ToWorkspace  VariableName=drie_l  SampleTime=0  SaveFormat=Matrix
      settings: Buffer=10000
  drie_r : ToWorkspace  VariableName=drie_r  SampleTime=0  SaveFormat=Matrix
      settings: Buffer=10000
  FCS_ae_rl_rie_drie_out : Outport  Port=1  InitialOutput=0
  wires:
  FCS_ae_rl_rie_drie/1 -> drie_l/1, RL2/1
  drie_actuator (with initial state)/1 -> FCS_ae_rl_rie_drie_out/1
  RL2/1 -> drie_r/1, drie_actuator (with initial state)/1

== system admire_linear_test/FCS_ae_rl/FCS_ae_rl_roe ==
  note: Level V
  FCS_ae_rl_roe_droe : Inport  Port=1  PortWidth=-1  SampleTime=-1  DataType=auto
      settings: SignalType=auto
  RL2 : RateLimiter  RisingSlewLimit=rlimit_oe+ddey_rate  FallingSlewLimit=-rlimit_oe-ddey_rate
  droe_actuator (with initial state) : simulink_extras/Additional Linear/Transfer Fcn (with initial states)  N=[1]  D="[0.05+ddey_bw  1]"  X0=[]
  droe_l : ToWorkspace  VariableName=droe_l  SampleTime=0  SaveFormat=Matrix
      settings: Buffer=10000
  droe_r : ToWorkspace  VariableName=droe_r  SampleTime=0  SaveFormat=Matrix
      settings: Buffer=10000
  FCS_ae_rl_roe_droe_out : Outport  Port=1  InitialOutput=0
  wires:
  droe_actuator (with initial state)/1 -> FCS_ae_rl_roe_droe_out/1
  FCS_ae_rl_roe_droe/1 -> droe_l/1, RL2/1
  RL2/1 -> droe_actuator (with initial state)/1, droe_r/1

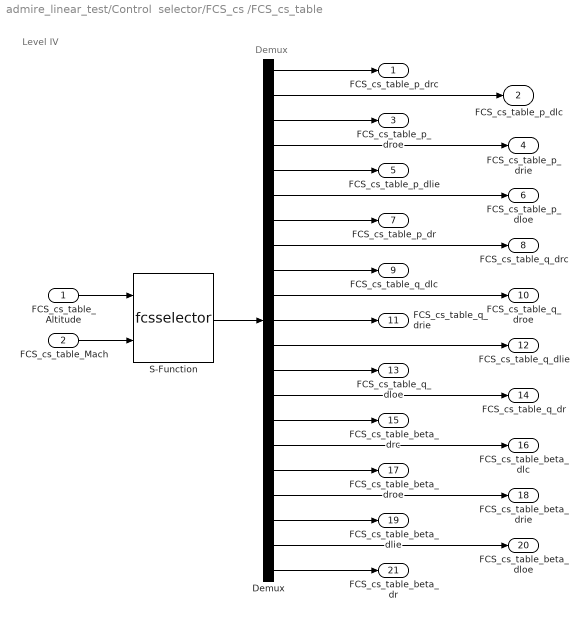
== system admire_linear_test/Control  selector/FCS_cs /FCS_cs_table ==
  note: Level IV
  note: Demux
  FCS_cs_table_Altitude : Inport  Port=1  PortWidth=-1  SampleTime=-1  DataType=auto
      settings: SignalType=auto
  FCS_cs_table_Mach : Inport  Port=2  PortWidth=-1  SampleTime=-1  DataType=auto
      settings: SignalType=auto
  Demux : Demux  Outputs=21
  S-Function : S-Function  FunctionName=fcsselector  PortCounts=[]  SFunctionModules=''
  FCS_cs_table_p_drc : Outport  Port=1
  FCS_cs_table_p_dlc : Outport  Port=2
  FCS_cs_table_p_droe : Outport  Port=3
  FCS_cs_table_p_drie : Outport  Port=4
  FCS_cs_table_p_dlie : Outport  Port=5
  FCS_cs_table_p_dloe : Outport  Port=6
  FCS_cs_table_p_dr : Outport  Port=7
  FCS_cs_table_q_drc : Outport  Port=8
  FCS_cs_table_q_dlc : Outport  Port=9
  FCS_cs_table_q_droe : Outport  Port=10
  FCS_cs_table_q_drie : Outport  Port=11
  FCS_cs_table_q_dlie : Outport  Port=12
  FCS_cs_table_q_dloe : Outport  Port=13
  FCS_cs_table_q_dr : Outport  Port=14
  FCS_cs_table_beta_drc : Outport  Port=15
  FCS_cs_table_beta_dlc : Outport  Port=16
  FCS_cs_table_beta_droe : Outport  Port=17
  FCS_cs_table_beta_drie : Outport  Port=18
  FCS_cs_table_beta_dlie : Outport  Port=19
  FCS_cs_table_beta_dloe : Outport  Port=20
  FCS_cs_table_beta_dr : Outport  Port=21
  wires:
  FCS_cs_table_Altitude/1 -> S-Function/1
  FCS_cs_table_Mach/1 -> S-Function/2
  S-Function/1 -> Demux/1
  Demux/3 -> FCS_cs_table_p_droe/1
  Demux/5 -> FCS_cs_table_p_dlie/1
  Demux/7 -> FCS_cs_table_p_dr/1
  Demux/9 -> FCS_cs_table_q_dlc/1
  Demux/11 -> FCS_cs_table_q_drie/1
  Demux/13 -> FCS_cs_table_q_dloe/1
  Demux/15 -> FCS_cs_table_beta_drc/1
  Demux/17 -> FCS_cs_table_beta_droe/1
  Demux/19 -> FCS_cs_table_beta_dlie/1
  Demux/21 -> FCS_cs_table_beta_dr/1
  Demux/2 -> FCS_cs_table_p_dlc/1
  Demux/4 -> FCS_cs_table_p_drie/1
  Demux/6 -> FCS_cs_table_p_dloe/1
  Demux/8 -> FCS_cs_table_q_drc/1
  Demux/10 -> FCS_cs_table_q_droe/1
  Demux/12 -> FCS_cs_table_q_dlie/1
  Demux/16 -> FCS_cs_table_beta_dlc/1
  Demux/18 -> FCS_cs_table_beta_drie/1
  Demux/20 -> FCS_cs_table_beta_dloe/1
  Demux/14 -> FCS_cs_table_q_dr/1
  Demux/1 -> FCS_cs_table_p_drc/1
